simulink model "PID_Controller_Sim"  (R2017b)
settings: Solver=VariableStepAuto  StartTime=0.0  StopTime=50  RelTol=1e-3
libraries: simulink x1
settings Model: Creator=Oguzhan  LastModifiedBy=Oguzhan

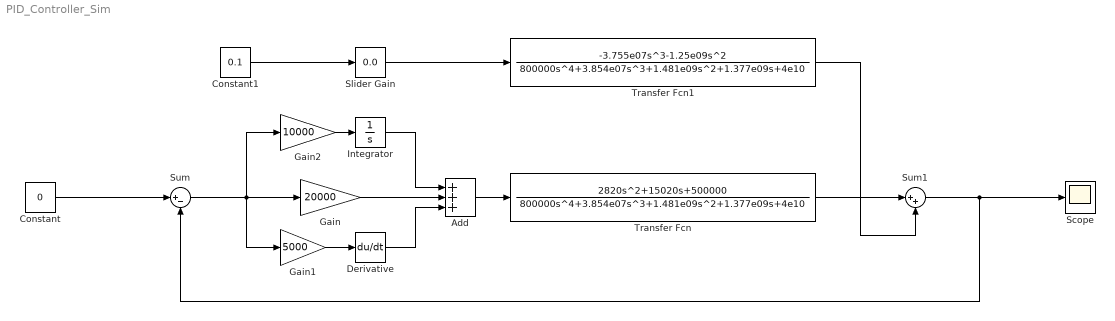
== system PID_Controller_Sim ==
  Add : Sum  Inputs=+++
  Constant : Constant  Value=0
  Constant1 : Constant  Value=0.1
  Derivative : Derivative
  Gain : Gain  Gain=20000
  Gain1 : Gain  Gain=5000
  Gain2 : Gain  Gain=10000
  Integrator : Integrator
  Scope : Scope
  Slider Gain : simulink/Math Operations/Slider Gain  gain=0.0  low=0  high=2
  Sum : Sum  Inputs=|+-
  Sum1 : Sum  Inputs=|++
  Transfer Fcn : TransferFcn  Numerator=[2820 15020 500000]  Denominator=[800000 3.854e07 1.481e09 1.377e09 4e10]
  Transfer Fcn1 : TransferFcn  Numerator=[-3.755e07 -1.25e09 0 0]  Denominator=[800000 3.854e07 1.481e09 1.377e09 4e10]
  wires:
  Sum/1 -> Gain2/1, Gain1/1, Gain/1
  Constant/1 -> Sum/1
  Constant1/1 -> Slider Gain/1
  Sum1/1 -> Scope/1, Sum/2
  Transfer Fcn/1 -> Sum1/1
  Transfer Fcn1/1 -> Sum1/2
  Gain1/1 -> Derivative/1
  Gain/1 -> Add/2
  Gain2/1 -> Integrator/1
  Derivative/1 -> Add/3
  Add/1 -> Transfer Fcn/1
  Integrator/1 -> Add/1
  Slider Gain/1 -> Transfer Fcn1/1
